simulink model "SimulinkModel_Template"  (Simulink 7.9)
settings: Solver=FixedStepDiscrete  SolverMode=MultiTasking  StartTime=0.0  StopTime=RunningTime  FixedStep=sample  RelTol=1e-3
values from neighbouring files (symbols this model uses):
  Integrator = CreateIntegrator(data(4), data(5), data(6), data2(1), data2(2))    [LoadConfiguration.m]    (also in ModelSetup.m = InitializeIntegrator(Integrator, Structure))
  NumFreeDOF = Structure.NumFreeDOF    [ModelSetup.m]
  RigidLinkMasterMatrix = Structure.RigidLinkMasterMatrix    [ModelSetup.m]
  RigidLinkNo = Structure.RigidLinkNo    [ModelSetup.m]
  RigidLinkNodeID = Structure.RigidLinkNodeID    [ModelSetup.m]
  RigidLinkSlaveMatrix = Structure.RigidLinkSlaveMatrix    [ModelSetup.m]
  sample = SampleRate/Integrator.Interpolations    [ModelSetup.m]
  SampleRate = Integrator.Timestep    [ModelSetup.m]
  Structure = CalculateMatrices(Structure, Elements, Integrator)    [ModelSetup.m]
undefined symbols (not defined in the file or in its folder): ElementsStruct
libraries: simulink x2
(part 2 of 2)

== matlab function Numerical Element Calculations ==
  data: Total_RF output double; NumFreeDOF parameter double; Displacement input double; Velocity input double; ElementsStruct parameter Bus: ElementStructBus; RigidLinkNo parameter double; RigidLinkNodeID parameter double; RigidLinkMasterMatrix parameter double; RigidLinkSlaveMatrix parameter double
%TODO: Els:3,5,7

% Get restoring force for each element
% Returns (6x1) restoring force vector of all elements in global coordinates
function Total_RF    = eml(NumFreeDOF, Displacement, Velocity, ElementsStruct, RigidLinkNo, RigidLinkNodeID, RigidLinkMasterMatrix, RigidLinkSlaveMatrix)
    % Store the Elements in memory
    persistent Elements;
    persistent TotalRF;
    if isempty(Elements)
        Elements = ElementsStruct;        
    end
    
    % Storage for the Global Restoring Force
    TotalRF = zeros(NumFreeDOF, 1);            
    
%Elements  %*s


%*e
                             
    Total_RF = TotalRF;
end


%%%%%%%%%%%%%%%%%%%%%%%%%%%%%%%%%%%%%%%%%%%%%%%%%%%%%%%%%%%%%%%%%%%%%%%%%%%
function TotalRF = AssembleElementGlobalRF6DOF(Element, ElementRF, TotalRF)
    % Assemble the structure restoring force vector based on the
    % degrees of freedom node locations.  
    ndof = 6;
    dof6 = zeros(6,1); 
    dof6(1,1)=Element.Nodes(1).UX;
    dof6(2,1)=Element.Nodes(1).UY;
    dof6(3,1)=Element.Nodes(1).THETA;
    dof6(4,1)=Element.Nodes(2).UX;
    dof6(5,1)=Element.Nodes(2).UY;
    dof6(6,1)=Element.Nodes(2).THETA;      

    % Add to the TotalRF
    for i=1:ndof
        if dof6(i,1) ~= -1
          TotalRF(dof6(i,1), 1) = ElementRF(i, 1) + TotalRF(dof6(i,1), 1);
        end
    end    
end

function TotalRF = AssembleElementGlobalRF9DOF(Element, ElementRF, TotalRF)
    % Assemble the structure restoring force vector based on the
    % degrees of freedom node locations.  
    ndof = 12;
    dof12 = zeros(12,1); 
    dof12(1,1)=Element.Nodes(1).UX;
    dof12(2,1)=Element.Nodes(1).UY;
    dof12(3,1)=Element.Nodes(1).THETA;
    dof12(4,1)=Element.Nodes(2).UX;
    dof12(5,1)=Element.Nodes(2).UY;
    dof12(6,1)=Element.Nodes(2).THETA;  
    dof12(7,1)=Element.Nodes(3).UX;
    dof12(8,1)=Element.Nodes(3).UY;
    dof12(9,1)=Element.Nodes(3).THETA;
    dof12(10,1)=Element.Nodes(4).UX;
    dof12(11,1)=Element.Nodes(4).UY;
    dof12(12,1)=Element.Nodes(4).THETA;

    % Add to the TotalRF
    for i=1:ndof
        if dof12(i,1) ~= -1
          TotalRF(dof12(i,1), 1) = ElementRF(i, 1) + TotalRF(dof12(i,1), 1);
        end
    end    
end

%% Element 1
function [Element, RestoringForce] = GetRestoringForce_Type1(Element, Displacement, RigidLinkNo, RigidLinkNodeID, RigidLinkMasterMatrix, RigidLinkSlaveMatrix)
    % Get distance between nodes
    X21 = Element.Nodes(2).Xcoord - Element.Nodes(1).Xcoord;
    Y21 = Element.Nodes(2).Ycoord - Element.Nodes(1).Ycoord;
    EL = sqrt(X21 * X21 + Y21 * Y21);
    EAL = Element.Material.E * Element.Area / EL;
    EIZL = Element.Material.E * Element.Inertia / EL;    
    % Calculation of density (the uniform load is only taken into account)
    SEP = zeros(6);
    SEP(1, 1) = EAL;
    SEP(1, 4) = -EAL;
    SEP(4, 4) = EAL;
    SEP(2, 2) = 12 * EIZL / EL ^ 2;
    SEP(2, 3) = 6 * EIZL / EL;
    SEP(2, 5) = -SEP(2, 2);
    SEP(2, 6) = SEP(2, 3);
    SEP(3, 3) = 4 * EIZL;
    SEP(3, 5) = -6 * EIZL / EL;
    SEP(3, 6) = 2 * EIZL;
    SEP(5, 5) = 12 * EIZL / EL ^ 2;
    SEP(5, 6) = -6 * EIZL / EL;
    SEP(6, 6) = 4 * EIZL;
    for i = 1:6
       for j = i:6
          SEP(j, i) = SEP(i, j);
       end
    end
    DCOS = zeros(3);
    DCOS(1, 1) = X21 / EL;
    DCOS(1, 2) = Y21 / EL;
    DCOS(1, 3) = 0;
    DCOS(2, 1) = -DCOS(1, 2);
    DCOS(2, 2) = DCOS(1, 1);
    DCOS(2, 3) = 0;
    DCOS(3, 1) = 0;
    DCOS(3, 2) = 0;
    DCOS(3, 3) = 1;
    ALMBDA = zeros(6);       
    for i = 1:2
       IK = 3 * (i - 1);
       for j = 1:3
          for k = 1:3
             ALMBDA(j + IK, k + IK) = DCOS(j, k);
          end
       end
    end
    SE = ALMBDA' * SEP * ALMBDA;
    % Create the displacement Ue (6x1) vector of the element in global coordinates
    Ue = zeros(6,1);
    dof = zeros(6,1);
    dof(1,1)=Element.Nodes(1).UX;
    dof(2,1)=Element.Nodes(1).UY;
    dof(3,1)=Element.Nodes(1).THETA;
    dof(4,1)=Element.Nodes(2).UX;
    dof(5,1)=Element.Nodes(2).UY;
    dof(6,1)=Element.Nodes(2).THETA;
    
    for i=1:6
        if dof(i,1) ~= -1
            Ue(i,1)=Displacement(dof(i,1),1);
        end
    end

    % Calculation Restoring Force, considering the Rigid Links if used
    if( RigidLinkNo )
        TR = RigidLinkTransformation2Nodes(Element.Nodes(1).ID, Element.Nodes(2).ID, RigidLinkNo, RigidLinkNodeID, RigidLinkMasterMatrix, RigidLinkSlaveMatrix);
        RestoringForce = TR' * SE * TR * Ue;  % (6x1) resisting force vector of element in global coordinates
    else        
        RestoringForce = SE * Ue;  % (6x1) resisting force vector of element in global coordinates
    end
end

%% Element 2
function [Element, RestoringForce] = GetRestoringForce_Type2(Element, Displacement, RigidLinkNo, RigidLinkNodeID, RigidLinkMasterMatrix, RigidLinkSlaveMatrix)
    % Preset arrays
    SE = zeros(6,6);
    SE(1, 1) = Element.Stiffness;
    SE(1, 4) = -Element.Stiffness;
    SE(4, 4) = Element.Stiffness;
    SE(4, 1) = SE(1,4);
    
    % Create the displacement Ue (6x1) vector of the element in global coordinates
    Ue = zeros(6,1);
    dof = zeros(6,1);
    dof(1,1)=Element.Nodes(1).UX;
    dof(2,1)=Element.Nodes(1).UY;
    dof(3,1)=Element.Nodes(1).THETA;
    dof(4,1)=Element.Nodes(2).UX;
    dof(5,1)=Element.Nodes(2).UY;
    dof(6,1)=Element.Nodes(2).THETA;
    
    for i=1:6
        if dof(i,1) ~= -1
            Ue(i,1)=Displacement(dof(i,1),1);
        end
    end

    % Calculation Restoring Force, considering the Rigid Links if used
    if( RigidLinkNo )
        TR = RigidLinkTransformation2Nodes(Element.Nodes(1).ID, Element.Nodes(2).ID, RigidLinkNo, RigidLinkNodeID, RigidLinkMasterMatrix, RigidLinkSlaveMatrix);
        RestoringForce = TR' * SE * TR * Ue;  % (6x1) resisting force vector of element in global coordinates
    else
%         if (RUNMODE_BIT)
%             RestoringForce = zeros(6,1);
%             RestoringForce(1,1) = Element2Input;
%             RestoringForce(4,1) = -Element2Input;
%         else
            RestoringForce = SE * Ue;  % (6x1) resisting force vector of element in global coordinates
%         end
    end    
end

%% Element 3

%% Element 4
function [Element, RestoringForce] = GetRestoringForce_Type4(Element, Displacement, RigidLinkNo, RigidLinkNodeID, RigidLinkMasterMatrix, RigidLinkSlaveMatrix)

    % element geometry       
    % element deformation % geometry restricted to 1,2 plane (x,y)
    dx = Element.xyj(1,1) - Element.xyi(1,1); 
    dy = Element.xyj(2,1) - Element.xyi(2,1);
    L = sqrt(dx*dx+dy*dy);
    dx = dx / L;
    dy = dy / L;

    % 6x6 transformation matrix from local to global coordiante
    apq  = zeros(6);
    apq(1,1) = dx; apq(2,2) = dx; apq(4,4) = dx; apq(5,5)= dx;
    apq(1,2) = dy; apq(2,1) =-dy; apq(4,5) = dy; apq(5,4)=-dy;
    apq(3,3) = 1.0; apq(6,6) =1.0;

    % element stiffness matrix in local coordinate
    SE = zeros(6,6);  
    SE(2, 2) = Element.K22;
    SE(2, 5) = Element.K25;
    SE(5, 2) = Element.K52;
    SE(5, 5) = Element.K55;
    % transformed element stiffness matrix in global coordinate
    SE = apq' * SE * apq;

    % Create the displacement Ue (6x1) vector of the element in global coordinates
    Ue = zeros(6,1);
    dof = zeros(6,1);
    dof(1,1)=Element.Nodes(1).UX;
    dof(2,1)=Element.Nodes(1).UY;
    dof(3,1)=Element.Nodes(1).THETA;
    dof(4,1)=Element.Nodes(2).UX;
    dof(5,1)=Element.Nodes(2).UY;
    dof(6,1)=Element.Nodes(2).THETA;

    for i=1:6
        if dof(i,1) ~= -1
            Ue(i,1) = Displacement(dof(i,1),1);
        end
    end
    
    % Calculation Restoring Force, considering the Rigid Links if used
    if( RigidLinkNo )
        TR = RigidLinkTransformation2Nodes(Element.Nodes(1).ID, Element.Nodes(2).ID, RigidLinkNo, RigidLinkNodeID, RigidLinkMasterMatrix, RigidLinkSlaveMatrix);
        RestoringForce = TR' * SE * TR * Ue;  % (6x1) resisting force vector of element in global coordinates
    else
        RestoringForce = SE * Ue;  % (6x1) resisting force vector of element in global coordinates
    end
end

%% Element 5

%% Element 6
function [Element,RestoringForce] = GetRestoringForce_Type6(Element, Displacement, RigidLinkNo, RigidLinkNodeID, RigidLinkMasterMatrix, RigidLinkSlaveMatrix)
    % Get the displacement Ue (6x1) vector of the element in global coordinates
    Ue = zeros(6,1);
    dof=zeros(6,1);
    dof(1,1)=Element.Nodes(1).UX;
    dof(2,1)=Element.Nodes(1).UY;
    dof(3,1)=Element.Nodes(1).THETA;
    dof(4,1)=Element.Nodes(2).UX;
    dof(5,1)=Element.Nodes(2).UY;
    dof(6,1)=Element.Nodes(2).THETA;
    for i=1:6
        if dof(i,1) ~= -1
            Ue(i,1)=Displacement(dof(i,1),1);
        end
    end

    % Calculation Restoring Force, considering the Rigid Links if used
    if( RigidLinkNo )
        TR = RigidLinkTransformation2Nodes(Element.Nodes(1).ID, Element.Nodes(2).ID, RigidLinkNo, RigidLinkNodeID, RigidLinkMasterMatrix, RigidLinkSlaveMatrix);        
        Ue = TR * Ue; 
    end       

    du=Ue-Element.Uprev;  % The incremental displacement vector du of the element in global coordinates 
    Element.Uprev=Ue; %Update Uprev of element for use in next state determination call

    % element deformation % geometry restricted to 1,2 plane (x,y)
    dx = Element.xyj(1,1) - Element.xyi(1,1); 
    dy = Element.xyj(2,1) - Element.xyi(2,1);
    L = sqrt(dx*dx+dy*dy);
    dx = dx / L;
    dy = dy / L;

    % Form transformation matrix from element in global coordinate to basic system
    avq  = [ -dy/L  dx/L  1  dy/L -dx/L  0;
           -dy/L  dx/L  0  dy/L -dx/L  1;
           -dx   -dy    0  dx    dy    0];

    % Incremental basic deformations
    dv = avq * du;        

    % Interpolation functions (B matrix) evaluated at integration points
    x  = ( Element.xi + 1 ) / 2;
    b1 = (6*x-4)/L;
    b2 = (6*x-2)/L;
    b3 = ones(size(x))/L;

    % Integrate basic force and basic stiffness matrix
    kb = zeros(3);
    s  = zeros(3,1);

    for i=1:length(Element.sections)

        % Form B matrix and compute section deformation
        B = [ b1(i) b2(i) 0; 0 0 b3(i) ];
        dvs = B * dv;  

        % Section state determination and update section state
        [ss ks Element.sections(i)] = SectionState( Element.sections(i), dvs );

        % Sum section term
        kb = kb + B'*ks*B * ( Element.wi(i) * L/2 );
        s  = s  + B'*ss   * ( Element.wi(i) * L/2 );

    end

    % Restoring force and stiffness matrix
    RestoringForce = avq' * s;

    if( RigidLinkNo )
        RestoringForce = TR' * RestoringForce;  
    end
end

%% Element 7

%% Element 8
function [Element,RestoringForce] = GetRestoringForce_Type8(Element, Displacement, Velocity, RigidLinkNo, RigidLinkNodeID, RigidLinkMasterMatrix, RigidLinkSlaveMatrix)
    % Get the displacement Ue (6x1) vector of the element in global coordinates
    Uev = zeros(6,1);
    Vev = zeros(6,1);
    dof=zeros(6,1);
    dof(1,1)=Element.Nodes(1).UX;
    dof(2,1)=Element.Nodes(1).UY;
    dof(3,1)=Element.Nodes(1).THETA;
    dof(4,1)=Element.Nodes(2).UX;
    dof(5,1)=Element.Nodes(2).UY;
    dof(6,1)=Element.Nodes(2).THETA;
    for i=1:6
        if dof(i,1) ~= -1
            Uev(i,1)=Displacement(dof(i,1),1);
            Vev(i,1)=Velocity(dof(i,1),1);        
        end
    end

    % Calculation Restoring Force, considering the Rigid Links if used
    if( RigidLinkNo )
        TR = RigidLinkTransformation2Nodes(Element.Nodes(1).ID, Element.Nodes(2).ID, RigidLinkNo, RigidLinkNodeID, RigidLinkMasterMatrix, RigidLinkSlaveMatrix);        
        Uev = TR * Uev; 
        Vev = TR * Vev; 
    end 

    % Deformation and velocity
    % if Element.dof ==1
    Ue = Uev(Element.dof,1)-Uev(Element.dof+3,1);
    Ve = Vev(Element.dof,1)-Vev(Element.dof+3,1);
    % elseif Element.dof ==2
    %     Ue = Uev(2,1)-Uev(5,1);
    %     Ve = Vev(2,1)-Vev(5,1);
    % else
    %     Ue = Uev(3,1)-Uev(6,1);
    %     Ve = Vev(3,1)-Vev(6,1);
    % end

    % Incremental displacement and velocity
    % the incremental deformation of the element 
    % Update max and min deformation history
    % Element.prop.Dmax= max(Ue,Element.prop.Dmax); 
    % Element.prop.Dmin= min(Ue,Element.prop.Dmin); 
    du = Ue - Element.Uprev;
    [Element.prop kt Fs] = MaterialState(du, Element.prop, Ve);

    RestoringForce=zeros(6,1);
    RestoringForce(Element.dof,1)   = Fs;
    RestoringForce(Element.dof+3,1) = -Fs;

    if( RigidLinkNo )
        RestoringForce = TR' * RestoringForce;  
    end

    % Update Uprev
    Element.Uprev=Ue; 
end


%% Element 9
function [Element,RestoringForce] = GetRestoringForce_Type9(Element, Displacement, RigidLinkNo, RigidLinkNodeID, RigidLinkMasterMatrix, RigidLinkSlaveMatrix)

%% Get the displacement Ue (12x1) vector of the element in global coordinates
ndof=12;  
Ue = zeros(ndof,1);
dof=zeros(ndof,1);
dof(1,1)=Element.Nodes(1).UX;
dof(2,1)=Element.Nodes(1).UY;
dof(3,1)=Element.Nodes(1).THETA;
dof(4,1)=Element.Nodes(2).UX;
dof(5,1)=Element.Nodes(2).UY;
dof(6,1)=Element.Nodes(2).THETA;
dof(7,1)=Element.Nodes(3).UX;
dof(8,1)=Element.Nodes(3).UY;
dof(9,1)=Element.Nodes(3).THETA;
dof(10,1)=Element.Nodes(4).UX;
dof(11,1)=Element.Nodes(4).UY;
dof(12,1)=Element.Nodes(4).THETA;

for i=1:ndof
    if dof(i,1) ~= -1
        Ue(i,1)=Displacement(dof(i,1),1);
    end
end

% Calculation Restoring Force, considering the Rigid Links if used
if( RigidLinkNo )
    TR = RigidLinkTransformation4Nodes(Element.Nodes(1).ID, Element.Nodes(2).ID, Element.Nodes(3).ID, Element.Nodes(4).ID, RigidLinkNo, RigidLinkNodeID, RigidLinkMasterMatrix, RigidLinkSlaveMatrix);        
    Ue = TR * Ue; 
end   

% The incremental displacement vector du of the element in global coordinates
% The element has 12 dofs
% Update Uprev of element for use in next state determination call
du=Ue-Element.Uprev;  
Element.Uprev=Ue; 

% transform global node displacement to basic deformation
v = Element.avq*Ue;

% compute element force
s = zeros(9,1); 

s(1) = Element.kb1*v(1);
s(2) = Element.kb2*v(2);
s(4) = Element.kb4*v(4);
s(5) = Element.kb5*v(5);
s(6) = Element.kb6*v(6);
s(7) = Element.kb7*v(7);
s(8) = Element.kb8*v(8);
s(9) = Element.kb9*v(9);

dv3 = Element.dx/Element.Width*du(10)-Element.dy/Element.Width*du(5)-Element.dx/Element.Width*du(4)+Element.dy/Element.Width*du(11)-Element.Height/Element.Width*Element.dx/Element.Width*du(2)...
    +Element.Height/Element.Width*Element.dy/Element.Width*du(1)+Element.Height/Element.Width*Element.dx/Element.Width*du(8)-Element.Height/Element.Width*Element.dy/Element.Width*du(7);

% compute shear deformation mode
[Element.ShearProp , tmp, s(3)]= MaterialState(dv3, Element.ShearProp, 0);

% Restoring force and stiffness matrix
RestoringForce = Element.avq' * s;

if( RigidLinkNo )
    RestoringForce = TR' * RestoringForce;  
end

% function [pro] = trilinear(dx, pro)
% 
% % calculate current deformation 
%     x = pro.xprev + dx; 
% 
% if pro.YieldCode == 0
% 
% 	pro.Fs1 = pro.Fs1+pro.K1*dx;
%     pro.Fs2 = pro.Fs2+pro.K2*dx;
% 	% if it is beyond elastic range, limit to yield force
% 	% and set m_nYieldCode to 1
% 	if pro.Fs1 > pro.Fy1
% 		
%         pro.Fs1 = pro.Fy1 ;
% 		pro.YieldCode = 1;
%         
%         if(pro.Fs2> pro.Fy2)
% 			pro.Fs2 = pro.Fy2 ;
% 		    pro.YieldCode = 2;
%         end
%     elseif pro.Fs1 < -pro.Fy1
% 		
%         pro.Fs1 = -pro.Fy1;
% 		pro.YieldCode = 1 ;
%        
% 		if pro.Fs2 < -pro.Fy2
% 			pro.Fs2 = - pro.Fy2 ;
% 		    pro.YieldCode = 2;
%         end
%     end
% % 1st post-yielding region    
% elseif pro.YieldCode == 1
%     
%     % assume spring2 remain elastic
%     pro.Fs2= pro.Fs2+pro.K2*dx;
%     
%     % keep loading
%     if pro.Fs1*dx > 0.
%         if pro.Fs2 > pro.Fy2
%             pro.Fs2 = pro.Fy2;
%             pro.YieldCode=2;            
%         elseif pro.Fs2 < -pro.Fy2
%             pro.Fs2 = -pro.Fy2;
%             pro.YieldCode=2;
%         end
%         % unloading
%     elseif pro.Fs1*dx < 0.
%         pro.Fs1= pro.Fs1 + pro.K1*dx;
%         pro.YieldCode = 0;
%         
%         if pro.Fs1 < -pro.Fy1 
%             pro.Fs1 = -pro.Fy1;
%             pro.YieldCode = 1;
%             if pro.Fs2 < -pro.Fy2
%                 pro.Fs2 = -pro.Fy2;
%                 pro.YieldCode = 2;
%             end
%         elseif pro.Fs1 > pro.Fy1
%             pro.Fs1 = pro.Fy1;
%             pro.YieldCode = 1;
%             if pro.Fs2 > pro.Fy2
%                 pro.Fs2 = pro.Fy2;
%                 pro.YieldCode = 2;
%             end
%         end
%     end
% elseif pro.YieldCode ==2
%     % unloading
% 	if (pro.Fs1*dx) < 0.
% 		pro.Fs1 = pro.Fs1 + pro.K1*dx;
% 		pro.Fs2 = pro.Fs2 + pro.K2*dx;
% 		pro.YieldCode = 0;
% 		
%         if pro.Fs1 < -pro.Fy1
%             pro.Fs1 = -pro.Fy1;
% 			pro.YieldCode = 1;
%             if pro.Fs2 < -pro.Fy2
% 				pro.Fs2 = -pro.Fy2;
% 				pro.YieldCode = 2;
%             end            
%         elseif pro.Fs1 > pro.Fy1
% 			pro.Fs1 = pro.Fy1;
% 			pro.YieldCode = 1;
%             if pro.Fs2> pro.Fy2
% 				pro.Fs2 = pro.Fy2;
% 				pro.YieldCode = 2;
% 			end
%         end
%     end
% end
% 
% pro.Fs = pro.Fs1 + pro.Fs2 + pro.K3*x;
% 
% % updata current state for next time step
% if pro.YieldCode == 0
%     pro.Kt = pro.K1 +pro.K2 +pro.K3;
% elseif pro.YieldCode == 1
%     pro.Kt = pro.K2 +pro.K3;    
% else
%     pro.Kt = pro.K3;
% end
% pro.xprev = x;

end
    

%%%%%%%%%%%%%%%%%%%%%%%%%%%%%%%%%%%%%%%%%%%%%%%%%%%%%%%%%%%%%%%%%%%%%%%%%%%
%%%%%%%%%%%%%%%%%%%%%%%%%%%% Helper Functions %%%%%%%%%%%%%%%%%%%%%%%%%%%%%
%%%%%%%%%%%%%%%%%%%%%%%%%%%%%%%%%%%%%%%%%%%%%%%%%%%%%%%%%%%%%%%%%%%%%%%%%%%

%% Rigid Link Tranformation Matrix Calculation for 2 Nodes, 6 DOF
function TR = RigidLinkTransformation2Nodes(Node1ID, Node2ID, RigidLinkNo, RigidLinkNodeID, RigidLinkMasterMatrix, RigidLinkSlaveMatrix)
    % Rigid Link Calculations
    TR = eye(6,6); % Transformation matrix for rigid link
    if( RigidLinkNo )    
        % Find the row with the slave node, if it exists in the element
        idx = 0;
        for kk = 1:RigidLinkNo
            if (RigidLinkNodeID(kk,2) == Node1ID)
                idx = kk;
                break;
            end
        end
        %idx=find(RigidLinkNodeID(:,2) == Node1ID); % find if a slave node exists in the element
        if ( idx )
            TL=CalculateRigidLinkTransformation(RigidLinkMasterMatrix(idx,2),RigidLinkMasterMatrix(idx,3),RigidLinkSlaveMatrix(idx,2),RigidLinkSlaveMatrix(idx,3));
            jjj = 1; % Node 1
            TR(3*(jjj-1)+1:3*jjj,3*(jjj-1)+1:3*jjj) = TL;
        end
        idx = 0;
        for kk = 1:RigidLinkNo
            if (RigidLinkNodeID(kk,2) == Node2ID)
                idx = kk;
                break;
            end
        end    
        %idx=find(RigidLinkNodeID(:,2) == Node2ID); % find if a slave node exists in the element
        if ( idx )
            TL=CalculateRigidLinkTransformation(RigidLinkMasterMatrix(idx,2),RigidLinkMasterMatrix(idx,3),RigidLinkSlaveMatrix(idx,2),RigidLinkSlaveMatrix(idx,3));            
            jjj = 2; % Node 2
            TR(3*(jjj-1)+1:3*jjj,3*(jjj-1)+1:3*jjj) = TL;
        end            
    end
end

%% Rigid Link Tranformation Matrix Calculation for 4 Nodes, 12 DOF
function TR = RigidLinkTransformation4Nodes(Node1ID, Node2ID, Node3ID, Node4ID, RigidLinkNo, RigidLinkNodeID, RigidLinkMasterMatrix, RigidLinkSlaveMatrix)
    % Rigid Link Calculations
    TR = eye(12,12); % Transformation matrix for rigid link
    if( RigidLinkNo )    
        % Find the row with the slave node, if it exists in the element
        idx = 0;
        for kk = 1:RigidLinkNo
            if (RigidLinkNodeID(kk,2) == Node1ID)
                idx = kk;
                break;
            end
        end
        %idx=find(RigidLinkNodeID(:,2) == Node1ID); % find if a slave node exists in the element
        if ( idx )
            TL=CalculateRigidLinkTransformation(RigidLinkMasterMatrix(idx,2),RigidLinkMasterMatrix(idx,3),RigidLinkSlaveMatrix(idx,2),RigidLinkSlaveMatrix(idx,3));
            jjj = 1; % Node 1
            TR(3*(jjj-1)+1:3*jjj,3*(jjj-1)+1:3*jjj) = TL;
        end
        idx = 0;
        for kk = 1:RigidLinkNo
            if (RigidLinkNodeID(kk,2) == Node2ID)
                idx = kk;
                break;
            end
        end    
        %idx=find(RigidLinkNodeID(:,2) == Node2ID); % find if a slave node exists in the element
        if ( idx )
            TL=CalculateRigidLinkTransformation(RigidLinkMasterMatrix(idx,2),RigidLinkMasterMatrix(idx,3),RigidLinkSlaveMatrix(idx,2),RigidLinkSlaveMatrix(idx,3));            
            jjj = 2; % Node 2
            TR(3*(jjj-1)+1:3*jjj,3*(jjj-1)+1:3*jjj) = TL;
        end                
        % Find the row with the slave node, if it exists in the element
        idx = 0;
        for kk = 1:RigidLinkNo
            if (RigidLinkNodeID(kk,2) == Node3ID)
                idx = kk;
                break;
            end
        end
        %idx=find(RigidLinkNodeID(:,2) == Node3ID); % find if a slave node exists in the element
        if ( idx )
            TL=CalculateRigidLinkTransformation(RigidLinkMasterMatrix(idx,2),RigidLinkMasterMatrix(idx,3),RigidLinkSlaveMatrix(idx,2),RigidLinkSlaveMatrix(idx,3));
            jjj = 3; % Node 3
            TR(3*(jjj-1)+1:3*jjj,3*(jjj-1)+1:3*jjj) = TL;
        end
        idx = 0;
        for kk = 1:RigidLinkNo
            if (RigidLinkNodeID(kk,2) == Node4ID)
                idx = kk;
                break;
            end
        end    
        %idx=find(RigidLinkNodeID(:,2) == Node4ID); % find if a slave node exists in the element
        if ( idx )
            TL=CalculateRigidLinkTransformation(RigidLinkMasterMatrix(idx,2),RigidLinkMasterMatrix(idx,3),RigidLinkSlaveMatrix(idx,2),RigidLinkSlaveMatrix(idx,3));            
            jjj = 4; % Node 4
            TR(3*(jjj-1)+1:3*jjj,3*(jjj-1)+1:3*jjj) = TL;
        end          
    end
end

%% Calculate Rigid Link Transformation
function TL = CalculateRigidLinkTransformation(MNXcoord, MNYcoord, SNXcoord, SNYcoord)
    X1 = MNXcoord; Y1 = MNYcoord;
    X2 = SNXcoord;  Y2 = SNYcoord;
    deltaX = X2 - X1;
    deltaY = Y2 - Y1;
    TL = [ 1 0 -deltaY;
           0 1  deltaX;
           0 0  1    ];
end

%% State determination for fiber section
function [ss, ks, sec] = SectionState( sec, dvs )
% For section sec undergoing a change
% in section deformation dvs=[curvature strain], compute
% section forces SS=[moment axial] and the 2x2 tangents
% section stiffness KS.
    ks = zeros(2,2);
    ss = zeros(2,1);  
    numfib = length(sec.fibers);

    % Loop over fibers
    for i=1:numfib
        yi   = sec.fibers(i).yi;
        area = sec.fibers(i).A;

        % Change in strain
        deps = yi * dvs(1:2);

        [sec.fibers(i).prop Et sc] = MaterialState(deps, sec.fibers(i).prop, 0 );        

        % Integration -- add contribution of fiber 
        % for 3D --- following codes need to be modified
        ks = ks + yi'*yi * (area*Et ); % may not need to do it
        ss = ss + yi'    * (area*sc);
    end
end

%% Material Section State
function [ mat Et sc] = MaterialState( dep, mat, vc)  
    %MATERIALSTATE Summary of this function goes here
    %   dep = incremental deformation at the current time step, except for
    %   Bouc-Wen model
    %   mat = material data structure
    %   vc  = 0 for other materials
    %       = current velocity for Bouc-Wen material
    %
    switch  mat.Type
        case 2
            mat = bilinearMat(dep, mat);
            Et = mat.Et;
            sc = mat.sc;
%         case 3
%             mat = hystereticMat(dep, mat);
%             Et = mat.Ttangent;
%             sc = mat.Cstress;
        case 4
            mat = BoucWen(dep, mat, vc);
            Et = mat.k;
            sc = mat.Qj;
        case 5
            mat = trilinear(dep, mat);
            Et = mat.Kt;
            sc = mat.Fs;
%         case 6
%             mat = SDegrading(dep, mat);
%             Et = mat.Ktan;
%             sc = mat.Fs;      
    %     case 7
    %         mat = ModifiedBW(dep, vc, mat);
    %         Et = mat.k;
    %         sc = mat.Qj;
        otherwise
            Et = 0;
            sc = 0;
    end
end

%% Bilinear Material Section State
function [mat] = bilinearMat(deps, mat )
    %	[mat]=BILINEARMAT(deps,mat) For strain increment deps
    %	and mat compute new properties for bilinear material.
    %	mat.SY, mat.E, mat.EP are the yield stress,
    %	first slop and second slope respectively.  materialProp.SC,
    %	mat.SB, materialSE are the current stress, back stress, and
    %	current strain, respectively. mat.ET is the current tangent modulus.

    % Material properties
    sigy = mat.sy;		% yield stress
    E    = mat.e;		% E
    Ep   = mat.ep;		% alpha*E

    % State from last converged load step
    sig  = mat.sc;		% stress
    sigb = mat.sb;		% backstress
    code = mat.cd;		% yield code
                        %	=0, elastic
                        %	=1, plastic

    if code==0 || ( code==1 && (sig-sigb)*deps < 0 )
        % Strain to plastic loading from elastic state
        deps1 = ( sign(deps) * sigy + sigb - sig ) / E;

        % Elastic
        sig  = sig + E * deps;
        Et   = E;
        code = 0;

        % Check if plasic loading from elastic state
        if abs(deps) > abs(deps1)
            sig  = sig  + ( Ep - E ) * ( deps - deps1 );
            sigb = sigb +   Ep       * ( deps - deps1 );
            Et   = Ep;
            code = 1;
        end

    else
        % Continue plastic loading
        sig  = sig  + Ep * deps;
        sigb = sigb + Ep * deps;
        Et   = Ep;
        code = 1;

    end

    % Return updated state. 
    mat.sc = sig;
    mat.sb = sigb;
    mat.cd = code;
    mat.es = mat.es + deps;	
    mat.Et = Et;
end   
% 
% %% Hysteretic Material Section State
% function [mat] = hystereticMat(deps, mat)   
%     mat.Tstrain = deps + mat.Cstrain;
% 
%     if (mat.TloadIndicator == 0 && mat.Tstrain == 0.0)
%         return ;
%     end
% 
%     mat.TrotMax = mat.CrotMax;
%     mat.TrotMin = mat.CrotMin;
%     mat.TenergyD = mat.CenergyD;
%     mat.TrotPu = mat.CrotPu;
%     mat.TrotNu = mat.CrotNu;
%     mat.TloadIndicator = mat.CloadIndicator;
% 
%     if (mat.TloadIndicator == 0)
%         if (deps < 0.0)
%             mat.TloadIndicator = 2;
%         else
%             mat.TloadIndicator = 1;
%         end
%     end
% 
%     if (mat.Tstrain >= mat.CrotMax) 
%         mat.TrotMax = mat.Tstrain;
%         mat.Ttangent= posEnvlpTangent(mat);
%         mat.Tstress = posEnvlpStress(mat,mat.Tstrain);
%         mat.TloadIndicator=1;
%     elseif (mat.Tstrain <= mat.CrotMin) 
%         mat.TrotMin = mat.Tstrain;
%         mat.Ttangent= negEnvlpTangent(mat);
%         mat.Tstress = negEnvlpStress(mat,mat.Tstrain);
%         mat.TloadIndicator=2;
%     else 
%         if (deps < 0.0)
%             mat=negativeIncrement(mat, deps);
%         elseif (deps > 0.0)
%             mat=positiveIncrement(mat, deps);
%         end
%     end
% 
%     mat.TenergyD = mat.CenergyD + 0.5*(mat.Tstress + mat.Cstress)*deps;
% 
%     % update the state for next time step
%     mat.CrotMax = mat.TrotMax;
%     mat.CrotMin = mat.TrotMin;
%     mat.CrotPu = mat.TrotPu;
%     mat.CrotNu = mat.TrotNu;
%     mat.CenergyD = mat.TenergyD;
%     mat.CloadIndicator = mat.TloadIndicator;
% 
%     mat.Cstress = mat.Tstress;
%     mat.Cstrain = mat.Tstrain;
% end
% 
% %% Negative Increment
% function [mat] = negativeIncrement(mat, deps)
%     kn = (mat.CrotMin/mat.rot1n)^mat.beta;
%     if kn < 1.0 
%         kn =  1.0; 
%     else kn = 1.0/kn; 
%     end;
% 
%     kp = (mat.CrotMax/mat.rot1p)^mat.beta;
%     if kp < 1.0 
%         kp =  1.0;
%     else kp = 1.0/kp; 
%     end;
% 
%     if (mat.TloadIndicator == 1) 
%         mat.TloadIndicator = 2;
%         if (mat.Cstress >= 0.0) 
% 
%             mat.TrotPu = mat.Cstrain - mat.Cstress/(mat.Eup* kp);
%             energy = mat.CenergyD -0.5*mat.Cstress/(mat.Eup* kp)*mat.Cstress;
%             damfc = 0.0;
% 
%             if (mat.CrotMax > mat.rot1p)
%                 damfc = mat.damfc1*(mat.CrotMax-mat.rot1p)/mat.rot1p + ...
%                     mat.damfc2* energy/ mat.energyA;
%             end
%             mat.TrotMin =  mat.CrotMin*(1.0+ damfc);		
%         end
%     end
% 
%     mat.TloadIndicator = 2;
% 
%     if mat.TrotMin >= mat.rot1n
%         mat.TrotMin =  mat.rot1n;
%     end
% 
%     minmom = negEnvlpStress(mat, mat.TrotMin);
%     rotlim = posEnvlpRotlim(mat);
%     if (rotlim < mat.TrotPu)
%         rotrel  = rotlim;
%     else
%         rotrel = mat.TrotPu;
%     end
% 
%     rotmp2 = mat.TrotMin - (1.0-mat.pinchY)*minmom/(mat.Eun*kn);
%     rotch  = rotrel + (rotmp2-rotrel)*mat.pinchX;     
% 
%     if (mat.Tstrain > mat.TrotPu) 
%         mat.Ttangent = mat.Eup*kp;
%         mat.Tstress = mat.Cstress + mat.Ttangent*deps;
%         if (mat.Tstress <= 0.0) 
%             mat.Tstress = 0.0;
%             mat.Ttangent = mat.Eup*1.0e-9;
%         end
%     elseif (mat.Tstrain <= mat.TrotPu && mat.Tstrain > rotch)
% 
%         if (mat.Tstrain >= rotrel) 
%             mat.Tstress = 0.0;
%             mat.Ttangent = mat.Eun*1.0e-9;
%         else 
%             mat.Ttangent = minmom *mat.pinchY/(rotch-rotrel);
%             tmpmo1 = mat.Cstress + mat.Eun* kn*deps;
%             tmpmo2 = (mat.Tstrain-rotrel)*mat.Ttangent;
%             if (tmpmo1 > tmpmo2) 
%                 mat.Tstress = tmpmo1;
%                 mat.Ttangent = mat.Eun*kn;
%             else
%                 mat.Tstress = tmpmo2;
%             end
%         end
%     else 
%         mat.Ttangent = (1.0-mat.pinchY)*minmom/(mat.TrotMin-rotch);
%         tmpmo1 = mat.Cstress + mat.Eun*kn*deps;
%         tmpmo2 = mat.pinchY*minmom + (mat.Tstrain-rotch)*mat.Ttangent;
%         if (tmpmo1 > tmpmo2)
%             mat.Tstress = tmpmo1;
%             mat.Ttangent = mat.Eun*kn;
%         else
%             mat.Tstress = tmpmo2;
%         end
%     end
% end
% 
% %% Positive Increment
% function [mat] = positiveIncrement(mat, deps)
%     kn = (mat.CrotMin/mat.rot1n)^mat.beta;
%     if (kn < 1.0) 
%         kn = 1.0;
%     else kn = 1.0/kn; 
%     end
% 
%     kp = (mat.CrotMax/mat.rot1p)^mat.beta;
%     if (kp < 1.0) 
%         kp = 1.0 ;
%     else kp =1.0/kp; 
%     end
% 
%     if mat.TloadIndicator == 2     
%         mat.TloadIndicator = 1;
% 
%         if (mat.Cstress <= 0.0)         
%             mat.TrotNu = mat.Cstrain - mat.Cstress/(mat.Eun*kn);
%             energy = mat.CenergyD - 0.5*mat.Cstress/(mat.Eun*kn)*mat.Cstress;
%             damfc = 0.0;
%             if (mat.CrotMin < mat.rot1n)
%                 damfc = mat.damfc2*energy/mat.energyA+ ...
%                     mat.damfc1*(mat.CrotMin-mat.rot1n)/mat.rot1n;
%             end
%             % update rotMax
%             mat.TrotMax = mat.CrotMax*(1.0+damfc);
%         end
%     end
% 
%     mat.TloadIndicator = 1;
% 
%     if (mat.TrotMax <= mat.rot1p) 
%         mat.TrotMax = mat.rot1p;
%     end
% 
%     maxmom = posEnvlpStress(mat, mat.TrotMax);
%     rotlim = negEnvlpRotlim(mat);
%     if (rotlim > mat.TrotNu) 
%         rotrel= rotlim;
%     else rotrel= mat.TrotNu; 
%     end;
% 
%     rotmp2 = mat.TrotMax - (1.0-mat.pinchY)*maxmom/(mat.Eup*kp);
%     rotch = rotrel + (rotmp2-rotrel)*mat.pinchX; 
% 
%     if (mat.Tstrain < mat.TrotNu)
%         mat.Ttangent = mat.Eun*kn;
%         mat.Tstress = mat.Cstress + mat.Ttangent*deps;
%         if (mat.Tstress >= 0.0) 
%             mat.Tstress = 0.0;
%             mat.Ttangent = mat.Eun*1.0e-9;
%         end
%     elseif (mat.Tstrain >= mat.TrotNu && mat.Tstrain < rotch) 
%         if (mat.Tstrain <= rotrel) 
%             mat.Tstress = 0.0;
%             mat.Ttangent = mat.Eup*1.0e-9;
%         else 
%             mat.Ttangent = maxmom*mat.pinchY/(rotch-rotrel);
%             tmpmo1 = mat.Cstress + mat.Eup*kp*deps;
%             tmpmo2 = (mat.Tstrain-rotrel)*mat.Ttangent;
%             if (tmpmo1 < tmpmo2) 
%                 mat.Tstress = tmpmo1;
%                 mat.Ttangent = mat.Eup*kp;
%             else
%                 mat.Tstress = tmpmo2;
%             end
%         end
%     else
%         mat.Ttangent = (1.0-mat.pinchY)*maxmom/(mat.TrotMax-rotch);
%         tmpmo1 = mat.Cstress + mat.Eup*kp*deps;
%         tmpmo2 = mat.pinchY*maxmom + (mat.Tstrain-rotch)*mat.Ttangent;
%         if (tmpmo1 < tmpmo2) 
%             mat.Tstress = tmpmo1;
%             mat.Ttangent = mat.Eup*kp;
%         else
%             mat.Tstress = tmpmo2;
%         end
%     end
% end
% 
% %% Positive Envelope Tangent
% function [posTangent] = posEnvlpTangent(mat)     
%     if (mat.Tstrain <= 0.0)
%         posTangent= mat.E1p*1.0e-9;
%     elseif (mat.Tstrain <= mat.rot1p)
%         posTangent= mat.E1p;
%     elseif (mat.Tstrain <= mat.rot2p)
%         posTangent= mat.E2p;
%     elseif (mat.Tstrain <= mat.rot3p || mat.E3p > 0.0)
%         posTangent= mat.E3p;
%     else
%         posTangent= mat.E1p*1.0e-9;
%     end
% end    
% 
% %% Negative Envelope Tangent
% function [negTangent] = negEnvlpTangent( mat)   
%     if (mat.Tstrain > 0.0)
%         negTangent= mat.E1n*1.0e-9;
%     elseif (mat.Tstrain >= mat.rot1n)
%         negTangent= mat.E1n;
%     elseif (mat.Tstrain >= mat.rot2n)
%         negTangent= mat.E2n;
%     elseif (mat.Tstrain >= mat.rot3n || mat.E3n > 0.0)
%         negTangent= mat.E3n;
%     else
%         negTangent= mat.E1n*1.0e-9;
%     end
% end
% 
% %% Positive Envelope Stress
% function [posStress] = posEnvlpStress(mat, strain)         
%     if (strain <= 0.0)
%         posStress = 0.0;
%     elseif (strain <= mat.rot1p)
%         posStress = mat.E1p*strain;
%     elseif (strain <= mat.rot2p)
%         posStress = mat.mom1p + mat.E2p*(strain-mat.rot1p);
%     elseif (strain <= mat.rot3p || mat.E3p > 0.0)
%         posStress = mat.mom2p + mat.E3p*(strain-mat.rot2p);
%     else
%         posStress = mat.mom3p;
%     end
% end
%       
% %% Negative Envelope Stress
% function [negStress] = negEnvlpStress(mat, strain)        
%     if (strain >= 0.0)
%         negStress = 0.0;
%     elseif (strain >= mat.rot1n)
%         negStress = mat.E1n*strain;
%     elseif (strain >= mat.rot2n)
%         negStress = mat.mom1n + mat.E2n*(strain-mat.rot1n);
%     elseif (strain >= mat.rot3n || mat.E3n > 0.0)
%         negStress = mat.mom2n + mat.E3n*(strain-mat.rot2n);
%     else
%         negStress = mat.mom3n;
%     end
% end
% 
% %% Negative Envelope Rotation Limit
% function [neglimit] = negEnvlpRotlim(mat)
%     neglimit =  -1.0e16;
% 
%     if (mat.CrotMin >= mat.rot1n) 
%         neglimit = -1.0e16; 
%     end;
%     if (mat.CrotMin < mat.rot1n && mat.CrotMin >= mat.rot2n && mat.E2n < 0.0)
%         neglimit = mat.rot1n - mat.mom1n/mat.E2n;
%     end;
%     if (mat.CrotMin < mat.rot2n && mat.E3n < 0.0) 
%         neglimit = mat.rot2n - mat.mom2n/mat.E3n;
%     end;
% 
%     if (neglimit ==  -1.0e16) 
%         neglimit = -1.0e16; 
%     elseif (negEnvlpStress(mat, neglimit) < 0)
%         neglimit = -1.0e16; 
%     end
% end
% 
% %% Positive Envelope Rotation Limit
% function [poslimit] = posEnvlpRotlim(mat)
%     poslimit =  1.0e16;
% 
%     if (mat.CrotMax <= mat.rot1p) 
%         poslimit =  1.0e16; 
%     end;
%     if (mat.CrotMax > mat.rot1p && mat.CrotMax <= mat.rot2p && mat.E2p < 0.0)
%         poslimit = mat.rot1p - mat.mom1p/mat.E2p;
%     end;
%     if (mat.CrotMax > mat.rot2p && mat.E3p < 0.0)
%         poslimit = mat.rot2p - mat.mom2p/mat.E3p;
%     end;
% 
%     if (poslimit == 1.0e16)
%         poslimit = 1.0e16;
%     elseif (posEnvlpStress(mat,poslimit) > 0)
%         poslimit = 1.0e16;
%     end
% end
% %%%%%%%%%%%%%%%%%%%% End of Hysteretic Material%% %%%%%%%%%%%%%%%%%%%%%%%%%
 
function [BW]= BoucWen( dx, BW, vcur)
    % ---------------------------------------------
    % x,v: displacement and velocity
    %   Q: restoring force
    %   z: hysteretic component
    %  zj: z in next step, i.e. z_i+1
    %  BW: numerous parameters for Bouc-Wen model
    %   i: step number

    xcur =  dx + BW.Uprev;
    % Fourth order R-K forward integration
    dz1 = dx*f(BW,vcur,BW.zj);
    dz2 = dx*f(BW,vcur,BW.zj+dz1/2);
    dz3 = dx*f(BW,vcur,BW.zj+dz2/2);
    dz4 = dx*f(BW,vcur,BW.zj+dz3);
    zj = BW.zj + (dz1+2*dz2+2*dz3+dz4)/6;

    umax=(abs(BW.Dmin)+ BW.Dmax)*0.5;    
    BW.k=BW.k1*exp(-umax/BW.uref) + BW.k2;    
    BW.Qj = BW.c*(abs(vcur)^BW.a)*sign(vcur) + BW.alpha*BW.k*xcur +...
        (1-BW.alpha)*BW.k*BW.uy*zj;

    % update deformation for next time step
    BW.Uprev = xcur;
    BW.Dmax= max(xcur,BW.Dmax); 
    BW.Dmin= min(xcur,BW.Dmin); 
    BW.zj =  zj;
end

function y=f(BW,v,z)
    % This function describes the nonlinear differential equation that governs
    % the hysteretic component, z.
    % The returned value is "dz/dx" or "z_dot/x_dot"
    y =(1/BW.uy)*(1-BW.beta*sign(v)*abs(z)^BW.n*sign(z)-BW.gamma1*abs(z)^BW.n);
end
%%%%%%%%%%%%%%%%%%% End of Bouc-Wen Model %%%%%%%%%%%%%%%%%%%%%%%% 

function [pro] = trilinear(dx, pro)
    % calculate current deformation 
        x = pro.xprev + dx; 

    if pro.YieldCode == 0

        pro.Fs1 = pro.Fs1+pro.K1*dx;
        pro.Fs2 = pro.Fs2+pro.K2*dx;
        % if it is beyond elastic range, limit to yield force
        % and set m_nYieldCode to 1
        if pro.Fs1 > pro.Fy1

            pro.Fs1 = pro.Fy1 ;
            pro.YieldCode = 1;

            if(pro.Fs2> pro.Fy2)
                pro.Fs2 = pro.Fy2 ;
                pro.YieldCode = 2;
            end
        elseif pro.Fs1 < -pro.Fy1

            pro.Fs1 = -pro.Fy1;
            pro.YieldCode = 1 ;

            if pro.Fs2 < -pro.Fy2
                pro.Fs2 = - pro.Fy2 ;
                pro.YieldCode = 2;
            end
        end
    % 1st post-yielding region    
    elseif pro.YieldCode == 1

        % assume spring2 remain elastic
        pro.Fs2= pro.Fs2+pro.K2*dx;

        % keep loading
        if pro.Fs1*dx > 0.
            if pro.Fs2 > pro.Fy2
                pro.Fs2 = pro.Fy2;
                pro.YieldCode=2;            
            elseif pro.Fs2 < -pro.Fy2
                pro.Fs2 = -pro.Fy2;
                pro.YieldCode=2;
            end
            % unloading
        elseif pro.Fs1*dx < 0.
            pro.Fs1= pro.Fs1 + pro.K1*dx;
            pro.YieldCode = 0;

            if pro.Fs1 < -pro.Fy1 
                pro.Fs1 = -pro.Fy1;
                pro.YieldCode = 1;
                if pro.Fs2 < -pro.Fy2
                    pro.Fs2 = -pro.Fy2;
                    pro.YieldCode = 2;
                end
            elseif pro.Fs1 > pro.Fy1
                pro.Fs1 = pro.Fy1;
                pro.YieldCode = 1;
                if pro.Fs2 > pro.Fy2
                    pro.Fs2 = pro.Fy2;
                    pro.YieldCode = 2;
                end
            end
        end
    elseif pro.YieldCode ==2
        % unloading
        if (pro.Fs1*dx) < 0.
            pro.Fs1 = pro.Fs1 + pro.K1*dx;
            pro.Fs2 = pro.Fs2 + pro.K2*dx;
            pro.YieldCode = 0;

            if pro.Fs1 < -pro.Fy1
                pro.Fs1 = -pro.Fy1;
                pro.YieldCode = 1;
                if pro.Fs2 < -pro.Fy2
                    pro.Fs2 = -pro.Fy2;
                    pro.YieldCode = 2;
                end            
            elseif pro.Fs1 > pro.Fy1
                pro.Fs1 = pro.Fy1;
                pro.YieldCode = 1;
                if pro.Fs2> pro.Fy2
                    pro.Fs2 = pro.Fy2;
                    pro.YieldCode = 2;
                end
            end
        end
    end

    pro.Fs = pro.Fs1 + pro.Fs2 + pro.K3*x;

    % updata current state for next time step
    if pro.YieldCode == 0
        pro.Kt = pro.K1 +pro.K2 +pro.K3;
    elseif pro.YieldCode == 1
        pro.Kt = pro.K2 +pro.K3;    
    else
        pro.Kt = pro.K3;
    end
    pro.xprev = x;
end
% 
% function [mat]= SDegrading(dx, mat)
%     %	[mat]=SDegrading(dx,mat) For incremental deformation, dx
%     %	and mat compute new properties for SDegrading material.
%     %	mat variables are defined in CreateMaterial.m
%     %   Line search algorithm is used to search for the current state
% 
%     % local variables
%     % accFac	: accumulated factor to trace out nonlinear path
%     % factor	: factor used to trace out nonlinear path
%     % fac	    : factor used to trace out nonlinear path
%     % dF        :
%     % uZero     :
%     % 
% 
%     dF = 0;	
%     accFac = 0.;
% 
%     while (accFac < 0.99999999)
% 
%         factor = 1.0 - accFac;
%         % current state is in elastic branch
%         if (mat.StateCode == 1)
%             % elastically loading
%             if (dx>0.)
%                 fac = (mat.Fyp-mat.Fs)/(mat.K1p*dx);
%                 if(fac<factor)
%                     factor = fac;
%                     mat.StateCode = 2;
%                 end
%             elseif (dx<0.)
%                 % in negative spring force
%                 fac = -mat.Fs/(mat.K1p*dx);
%                 % change in state
%                 if (fac < factor)
%                     factor = fac;
%                     mat.StateCode = -1;
%                 end
%             end
%             dF = mat.K1p*dx;
% 
%         elseif (mat.StateCode == -1)
% 
%             % elastically loading
%             if (dx<0.)
%                 fac = (mat.Fyn-mat.Fs)/(mat.K1n*dx);
%                 if(fac<factor)
%                     factor = fac;
%                     mat.StateCode = -2;
%                 end
%                 % elastically unloading
%             elseif (dx>0.)
%                 % in negative spring force
%                 fac = -mat.Fs/(mat.K1n*dx);
%                 % change in state
%                 if(fac < factor)
%                     factor = fac;
%                     mat.StateCode = 1;
%                 end
%             end
%             dF = mat.K1n*dx;
%             % current state is in yielding branch
%         elseif (mat.StateCode == 2)
% 
%             % elastically unloading along the line 5
%             if(dx < 0.)
%                 factor =0.;
%                 mat.StateCode = 5;
%                 mat.Umax = mat.Us;
%                 mat.Fmax = mat.Fs;
%                 % continue to yield
%             elseif (dx > 0.)
%                 fac = (mat.Uup - mat.Us) / dx;
%                 if(fac<factor)
%                     factor = fac;
%                     mat.StateCode  = 3;
%                 end
%                 dF = mat.K2p*dx;
%            %     mat.Fmax = mat.Fs;
%            %     mat.Umax = mat.Us;
%             end
% 
%         elseif (mat.StateCode == -2)
% 
%             % elastically unloading along the line 5
%             if (dx > 0.)
%                 factor =0.;
%                 mat.StateCode = -5;
%                 mat.Umin = mat.Us;
%                 mat.Fmin = mat.Fs;
%                 % continue to yield
%             elseif (dx <0.)
%                 fac = (mat.Uun - mat.Us) / dx;
%                 if(fac<factor)
%                     factor = fac;
%                     mat.StateCode = -3;
%                 end
%                 dF = mat.K2n*dx;
%         %        mat.Fmin = mat.Fs;
%         %        mat.Umin = mat.Us;
%             end
%             % current state is in descending branch
%         elseif ( mat.StateCode == 3)
% 
%            %	 elastically unloading
%             if (dx < 0.)
%                 factor =0.;
%                 mat.StateCode = 5;
%                 % in positive spring force
%                 mat.Umax = mat.Us;
%                 mat.Fmax = mat.Fs;
%                 % continue to yield
%             elseif (dx > 0.)
%                 % in positive spring force
%                 fac = (mat.Frp-mat.Fs) /(mat.K3p*dx);
%                 % change in state
%                 if (fac<factor)
%                     factor = fac;
%                     mat.StateCode  = 4;
%                 end
%                 dF = mat.K3p*dx;
%             end
%         elseif ( mat.StateCode == -3)
% 
%              % elastically unloading
%             if (dx > 0.)
%                 factor =0.;
%                 mat.StateCode = -5;
%                 % in positive spring force
%                 mat.Umin = mat.Us;
%                 mat.Fmin = mat.Fs;
%                 % continue to yield
%             elseif (dx < 0.)
%                 % in positive spring force
%                 fac = (mat.Frn-mat.Fs) /(mat.K3n*dx);
%                 % change in state
%                 if (fac<factor)
%                     factor = fac;
%                     mat.StateCode  = -4;
%                 end
%                 dF = mat.K3n*dx;
%             end
%         elseif (mat.StateCode == 4)
% 
%             % elastically unloading
%             if(dx < 0.)
%                 factor =0.;
%                 mat.StateCode = 5;
%                 mat.Umax = mat.Us;
%                 mat.Fmax = mat.Fs;
%             elseif (dx > 0.)
%                 dF = mat.K4p*dx;
%             end
% 
%         elseif (mat.StateCode == -4)
% 
%             % elastically unloading
%             if (dx > 0.)
%                 factor =0.;
%                 mat.StateCode = -5;
%                 mat.Umin = mat.Us;
%                 mat.Fmin = mat.Fs;
%             elseif (dx < 0.)
%                 dF = mat.K4n*dx;
%             end
%             % unloading branch
%         elseif (mat.StateCode == 5)
% 
%             % elastically reloading branch
%             if ( dx > 0.)
%                 fac = (mat.Fmax - mat.Fs)/(mat.K1p*dx);
%                 if(fac < factor)
%                     % update factor
%                     factor = fac;
%                     if mat.Umax >= mat.Urp
%                         mat.StateCode = 4;
%                     elseif mat.Umax >= mat.Uup
%                         mat.StateCode = 3;                    
%                     elseif mat.Umax >= mat.Uyp
%                         mat.StateCode = 2;
%                     end
%                 end
%             elseif ( dx < 0.)
%                 fac =  -mat.Fs/(mat.K1p*dx);
%                 if(fac < factor)
%                     factor = fac;
%                     mat.StateCode = -6;
%                     uZero = mat.Us+factor*dx;
%                     mat.K6	= mat.Fmin/(mat.Umin-uZero);
%                 end
%             end
%             dF = mat.K1p*dx;
% 
%         elseif (mat.StateCode == -5)
% 
%             % elastically reloading branch
%             if( dx < 0.)
%                 fac = (mat.Fmin - mat.Fs)/(mat.K1n*dx);
%                 if (fac < factor)
%                     % update factor
%                     factor = fac;
%                     if mat.Umin <= -mat.Urn
%                         mat.StateCode = -4;
%                     elseif mat.Umin <= -mat.Uun
%                         mat.StateCode = -3;                    
%                     elseif mat.Umin <= -mat.Uyn
%                         mat.StateCode = -2;
%                     end
%                 end
%             elseif ( dx > 0.)
%                 fac = -mat.Fs/(mat.K1n*dx);
%                 if (fac < factor)
%                     factor = fac;
%                     mat.StateCode = 6;
%                     uZero = mat.Us+factor*dx;
%                     mat.K6	= mat.Fmax/(mat.Umax-uZero);
%                 end
%             end
%             dF = mat.K1n*dx;
% 
%             % current state is in shooting branch
%         elseif (mat.StateCode == 6)
% 
%             % elastically unloading
%             if (dx< 0.)
%                 factor = 0.;
%                 mat.StateCode = 7;
%                 mat.Ftem = mat.Fs;
%                 mat.Utem = mat.Us;
%                 % continue to shoot
%             elseif (dx> 0.)
%                 fac = (mat.Umax-mat.Us)/dx;
%                 if (fac<factor)
%                     factor = fac;
%                     if mat.Umax >= mat.Urp
%                         mat.StateCode = 4;
%                     elseif mat.Umax >= mat.Uup
%                         mat.StateCode = 3;                    
%                     elseif mat.Umax >= mat.Uyp
%                         mat.StateCode = 2;
%                     end
%                 end
%                 dF = mat.K6*dx;
%             end
% 
%         elseif (mat.StateCode == -6)
% 
%             % elastically unloading
%             if(dx>0.)
%                 factor = 0.;
%                 mat.StateCode = -7;
%                 mat.Ftem = mat.Fs;
%                 mat.Utem = mat.Us;
%             elseif (dx<0.)
%                 fac = (mat.Umin-mat.Us)/dx;
%                 if (fac< factor)
%                     factor= fac;
%                     if mat.Umin <= mat.Urn
%                         mat.StateCode = -4;
%                     elseif mat.Umin <= mat.Uun
%                         mat.StateCode = -3;                    
%                     elseif mat.Umin <= mat.Uyn
%                         mat.StateCode = -2;
%                     end
%                 end
%                 dF = mat.K6*dx;
%             end
% 
%             % unloading branch off shooting branch
%         elseif (mat.StateCode == 7)
% 
%             % elastically reloads
%             if(dx>0.)
%                 fac = (mat.Utem -mat.Us)/dx;
%                 if (fac < factor)
%                     factor  = fac;
%                     mat.StateCode  = 6;
%                 end
%                 % continue unloading elastically
%             elseif (dx<0.)
%                 fac = -mat.Fs/(mat.K1p*dx);
%                 % change in state
%                 if (fac < factor)
%                     factor = fac;
%                     mat.StateCode =-6;
%                     % update stiffness in line 6
%                     uZero = mat.Us + factor*dx; 
%                     mat.K6 = mat.Fmin/(mat.Umin-uZero);
%                 end
%             end
%             dF = mat.K1p*dx;
% 
%         elseif (mat.StateCode == -7)
% 
%             % elastically reloads
%             if(dx<0.)
%                 fac = (mat.Utem -mat.Us)/dx;
%                 if(fac < factor)
%                     factor  = fac;
%                     mat.StateCode  = -6;
%                 end
%                 % continue unloading elastically
%             elseif (dx>0.)
%                 fac = -mat.Fs/(mat.K1n*dx);
%                 % change in state
%                 if (fac < factor)
%                     factor = fac;
%                     mat.StateCode =6;
%                     % update stiffness in line 6
%                     uZero =mat.Us + factor*dx;
%                     mat.K6 = mat.Fmax/(mat.Umax-uZero);
%                 end
%             end
%             dF = mat.K1n*dx;
% 
%         else
%             % do nothing
%         end
% 
%         % update state
%         mat.Us = mat.Us + factor*dx;
%         mat.Fs= mat.Fs + factor*dF;
% 
%         accFac = accFac+factor;
%     end
% 
%     % update stiffness at the current state
%     if mat.StateCode == 1
%         mat.Ktan = mat.K1p;
%     elseif mat.StateCode == -1
%         mat.Ktan = mat.K1n;    
%     elseif mat.StateCode == 2
%         mat.Ktan = mat.K2p;
%     elseif mat.StateCode == -2
%         mat.Ktan = mat.K2n;    
%     elseif (mat.StateCode) == 3
%         mat.Ktan = mat.K3p;
%     elseif (mat.StateCode) == -3
%         mat.Ktan = mat.K3n;
%     elseif (mat.StateCode) == 4
%         mat.Ktan = mat.K4p;
%     elseif (mat.StateCode) == -4
%         mat.Ktan = mat.K4n;
%     elseif abs(mat.StateCode) == 6
%         mat.Ktan = mat.K6;
%     end
% end
% 
% % %%%%%%%%%%%%%%%%%%%%%%%%%%%%%%%%%%%%%%%%%%%%%%%%%%%%%%%%%%%%%%%%%%%%%%
% % function [mat]= ModifiedBW(dx, v, mat)
% % % Modified Bouc-Wen model hysteresis model
% % % C. P. Heine (2001). Simulated response of degrading hysteretic joints with slack behaviour. PhD dissertation. 
% % % Virginial Polytechnic Institute and State University. Blacksburg, Virginia 
% % % URL: http://scholar.lib.vt.edu/theses/available/etd-08092001-100756
% % % Employ the 4th order Runge-Kutta forward integration
% % 
% % % ---------------------------------------------
% % % x,v: displacement and velocity
% % %   Q: restoring force
% % %   z: hysteretic component
% % %  zj: z in next step, i.e. z_i+1
% % %  MBW: numerous parameters for Modified Bouc-Wen model
% % %   i: step number
% % 
% %     xcur = dx+ mat.UPrev;
% %     
% % % Fourth order R-K forward integration
% %     dz1 = dx*G(mat, v, mat.z, mat.e);
% %     de1 = dx*F(mat, mat.z);
% %     dz2 = dx*G(mat, v, mat.z+dz1/2, mat.e +de1/2);
% %     de2 = dx*F(mat, mat.z +dz1/2);
% %     dz3 = dx*G(mat, v, mat.z+dz2/2, mat.e +de2/2);
% %     de3 = dx*F(mat, mat.z +dz2/2);
% %     dz4 = dx*G(mat, v, mat.z+dz3, mat.e +de3);
% %     de4 = dx*F(mat, mat.z +dz3);
% %     
% %     zj = mat.z + (dz1+2*dz2+2*dz3+dz4)/6;
% %     ej = mat.e + (de1+2*de2+2*de3+de4)/6;
% %     s = Slack(mat, zj); % slack growth
% % 
% % BW.Qj = s*mat.alpha*mat.k*xcur  + (1-mat.alpha)*mat.k*zj;
% % 
% % % update state 
% % mat.UPrev = xcur;
% % mat.Umax= max(xcur ,mat.Umax); 
% % mat.Umin= min(xcur ,mat.Umin); 
% % mat.absUmax=max([(abs(mat.Umin)), mat.Umax]);
% % mat.e = ej;
% % mat.z = zj;
% % 
% % function z = G(mat, v, z, eps)
% % % This function describes the nonlinear differential equation that governs
% % % the hysteretic component, z.
% % % The returned value is "dz/dx" or "z_dot/x_dot"
% % eta  = ETA(mat, eps);
% % nu   = NU(mat, eps);
% % h    = H(mat, z);
% % a    = A(mat, eps); 
% % z  = h*(1/eta)*(a-nu*(mat.beta*sign(v)*abs(z)^mat.n*sign(z)-mat.gamma1*abs(z)^mat.n));
% % 
% % function de_du = F(mat, z)
% % de_du = (1-mat.alpha)*mat.k*z;
% % 
% % function h = H(mat, z)
% % h = 1-mat.Xi*exp(-z^2./(mat.psi0+ mat.delta_psi*abs(mat.absUmax))^2.);
% % 
% % function eta =ETA(mat, eps)
% % eta = 1+ mat.delta_eta*eps;
% % 
% % function nu = NU(mat, eps)
% % nu = 1+ mat.delta_nu*eps;
% % 
% % function a = A(mat, eps)
% % a = mat.a0 - mat.delta_a*eps;
% % 
% % function s = Slack(mat, z)
% % s = 1 - exp(-z^2./(mat.psi0+ mat.delta_psi*abs(mat.absUmax))^2.);
% % 
% 
%
